simulink model "DPT"  (R2023a)
settings: Solver=VariableStepAuto  StartTime=0.0  StopTime=10.0  RelTol=1e-3
values from neighbouring files (symbols this model uses):
  C_m = 1.3    [untitled.m]
  C_w = 3.15    [untitled.m]
  J_dv = 7 * 10^-6    (= 7e-06)    [untitled.m]
  L_a = 0.0015    [untitled.m]
  L_ov = 0.013    [untitled.m]
  R_a = 8    [untitled.m]
  U_c = 5    [untitled.m]
settings Model: Creator=tatyn  LastModifiedBy=tatyn

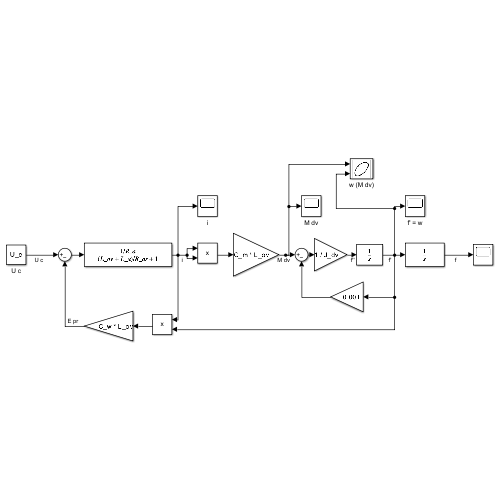
[thumbnail: Simulink's stored preview of the top-level diagram]
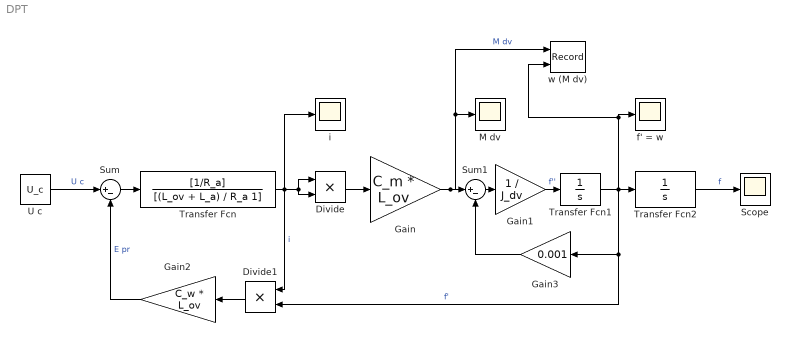
== system DPT ==
  Divide : Product  Inputs=**
  Divide1 : Product  Inputs=**
  Gain : Gain  Gain=C_m * L_ov
  Gain1 : Gain  Gain=1 / J_dv
  Gain2 : Gain  Gain=C_w * L_ov
  Gain3 : Gain  Gain=0.001
  Scope : Scope
  Sum : Sum  Inputs=|+-
  Sum1 : Sum  Inputs=|+-
  Transfer Fcn : TransferFcn  Numerator=[1/R_a]  Denominator=[(L_ov + L_a) / R_a 1]
  Transfer Fcn1 : TransferFcn  Denominator=[1 0]
  Transfer Fcn2 : TransferFcn  Denominator=[1 0]
  U c : Constant  Value=U_c
  f' = w : Scope
  i : Scope
  w (M dv) : Record  FileSettingsInternal="{\"entries\":[{\"content\":{\"excelSettings\":{\"content\":{},\"type\":\"Streamout.ExcelSettings\"}},\"type\":\"Streamout.FileSettingStorage\",\"uuid\":\"ea350697-1ea9-45a1-a5f9-1f43d1747978\"}],\"packageUris\":[\"http://schema.mathworks.com/mf0/streamout_blocks/R2020a\"],\"version\":\"1.0\"}"  Layout=[1 1]  SignalsInternal="{\"entries\":[{\"content\":{\"signals\":[{\"content\":{\"blockPath\":[\"DPT/w (M dv)\"],\"dimensions\":[1],\"domain\":\"DPT/w (M dv)\",\"lineColor\":\"#edb120\",\"port\":1,\"sid\":[\"\"],\"signalID\":19,\"signalName\":\"M dv\"},\"type\":\"RecordBlkView.Signal\",\"uuid\":\"5ea0c725-af79-49e1-95b0-6736d0a93210\"},{\"content\":{\"blockPath\":[\"DPT/w (M dv)\"],\"dimensions\":[1],\"domain\":\"DPT/w (M dv)\",\"lineColor\":\"#7e2f8e\",\"port\":2,\"sid\":[\"\"],\"signalID\":23,\"signalName\":\"f'\"},\"type\":\"RecordBlkView.Signal\",\"uuid\":\"cd4b2f48-d550-49c1-b88d-d036d331908d\"}]},\"type\":\"RecordBlkView.InputSignals\",\"uuid\":\"08c1e611-8748-4c8f-98ea-9f5ebe998b1e\"}],\"packageUris\":[\"http://schema.mathworks.com/mf0/streamout_blocks/R2020a\"],\"version\":\"1.0\"}"  VisualizationBindings="{\"xyplotplugin\":{\"info\":[{\"series\":[],\"subplotID\":1}]}}"  CompatibilityTag=XY
  М dv : Scope
  wires:
  U c/1 -> Sum/1  "U c"
  Sum/1 -> Transfer Fcn/1
  Divide/1 -> Gain/1
  Transfer Fcn/1 -> Divide/2, Divide/1, Divide1/1, i/1  "i"
  Gain/1 -> w (M dv)/1, М dv/1, Sum1/1  "M dv"
  Gain1/1 -> Transfer Fcn1/1  "f''"
  Transfer Fcn1/1 -> w (M dv)/2, f' = w/1, Gain3/1, Divide1/2, Transfer Fcn2/1  "f'"
  Transfer Fcn2/1 -> Scope/1  "f"
  Divide1/1 -> Gain2/1
  Gain2/1 -> Sum/2  "Е pr"
  Sum1/1 -> Gain1/1
  Gain3/1 -> Sum1/2
